simulink model "bp"  (Simulink 7.1)
settings: Solver=ode5  StartTime=0.0  StopTime=170.0  FixedStep=0.1  RelTol=1e-3  AbsTol=1e-3
undefined symbols (not defined in the file): sfunyst
libraries: fuzblock x3
settings Model: Creator=Slavi  LastModifiedBy=Slavi  BufferReuse=off
settings DataIOCC: LimitDataPoints=off  SaveOutput=off  SaveTime=off  SignalLoggingName=sigsOut
settings OptimizationCC: BlockReduction=off  BooleanDataType=off  OptimizeBlockIOStorage=off  BufferReuse=off  ExpressionFolding=off  LocalBlockOutputs=off
settings DebuggingCC: SaveWithParameterizedLinksMsg=none  SignalResolutionControl=TryResolveAllWithWarning  SolverPrmCheckMsg=none  MultiTaskDSMMsg=warning  MultiTaskCondExecSysMsg=none  StrictBusMsg=None
settings HardwareCC: TargetUnknown=on
settings RTWCC: IncludeERTFirstTime=on

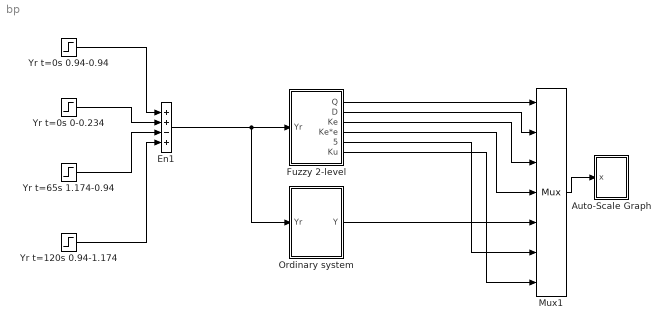
== system bp ==
  Auto-Scale Graph : Subsystem  mask(Storage scope.){@1=170, @2=0, @3=2, @4=20000, @5='r-/m-/b-/g-/k-/r-/b:', @6=.1}
      mask prompts: @1 "Initial Time Range:"; @2 "Initial y-min:"; @3 "Initial y-max:"; @4 "Storage pts.:"; @5 "Line type (rgbw-.:xo):"; @6 "Sample time:"
      mask help:
      | Storage scope using MATLAB graph window.
      | Enter plotting ranges and line type.
      mask init:
      | npts = @4; color = @5; ax = [0, @1, @2, @3]; dt=@6;
      mask Help: Uses MATLAB's graph window.\nUse only one block per system.\nLine type must be in quotes.\nSee the M-file sfunyst.m.
      mask Display: plot(0,0,100,100,[83,76,63,52,42,38,28,16,11,84,11,11,11,90,90,11],[75,58,47,54,72,80,84,74,65,65,65,90,40,40,90,90])
  En1 : Sum  Inputs=++-+  OutDataType=sfix(16)  OutScaling=2^0  SaturateOnIntegerOverflow=on  InputSameDT=on  OutDataTypeStr=Inherit: Same as first input
  Fuzzy 2-level : Subsystem
  Mux1 : Mux  Inputs=7
  Ordinary system : Subsystem
  Yr t=0s 0-0.234 : Step  Time=0  After=0.234  SampleTime=0.1
  Yr t=0s 0.94-0.94 : Step  Time=0  Before=0.94  After=0.94  SampleTime=0.1
  Yr t=120s 0.94-1.174 : Step  Time=120  After=0.234  SampleTime=0.1
  Yr t=65s 1.174-0.94 : Step  Time=65  After=0.234  SampleTime=0.1
  wires:
  Mux1/1 -> Auto-Scale Graph/1(x)
  Yr t=0s 0.94-0.94/1 -> En1/1
  En1/1 -> Fuzzy 2-level/1(Yr), Ordinary system/1(Yr)
  Fuzzy 2-level/1(Q) -> Mux1/1
  Fuzzy 2-level/2(D) -> Mux1/2
  Fuzzy 2-level/3(Ke) -> Mux1/3
  Ordinary system/1(Y) -> Mux1/5
  Fuzzy 2-level/4(Ke*e) -> Mux1/4
  Fuzzy 2-level/5("  Sum(e^2) ") -> Mux1/6
  Fuzzy 2-level/6(Ku) -> Mux1/7
  Yr t=0s 0-0.234/1 -> En1/2
  Yr t=65s 1.174-0.94/1 -> En1/3
  Yr t=120s 0.94-1.174/1 -> En1/4

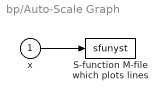
== system bp/Auto-Scale Graph ==
  x : Inport  OutDataType=sfix(16)  OutScaling=2^0
  "S-function M-file which plots lines " : S-Function  LoadFcn=sfunyst([],[],[],'LoadBlock')  FunctionName=sfunyst  Parameters=ax, color, npts, dt  EnableBusSupport=off
      settings: CopyFcn=sfunyst([],[],[],'CopyBlock')  DeleteFcn=sfunyst([],[],[],'DeleteBlock')
  wires:
  x/1 -> "S-function M-file which plots lines "/1

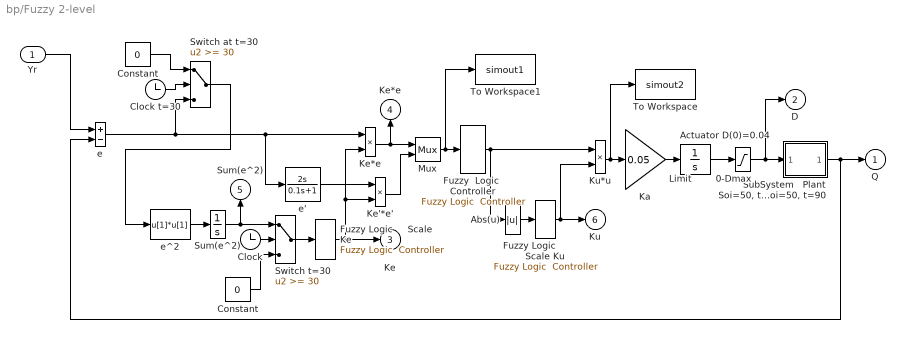
== system bp/Fuzzy 2-level ==
  Yr : Inport  SampleTime=0.5  OutDataType=sfix(16)  OutScaling=2^0
  "        Fuzzy Logic            Scale Ku" : fuzblock/Fuzzy Logic  Controller  SystemSampleTime=-1  fis=supervisor_razmit.fis
  "      Limit        0-Dmax" : Saturate  UpperLimit=0.3  LowerLimit=0
  "  Fuzzy Logic     Scale Ke" : fuzblock/Fuzzy Logic  Controller  SystemSampleTime=-1  fis=supervisor_razmit.fis
  "Abs(u) " : Abs  SaturateOnIntegerOverflow=on
  Actuator D(0)=0.04 : Integrator  InitialCondition=0.04
  Clock t=30 : Clock
      settings: Decimation=30
  "Clock  " : Clock
      settings: Decimation=30
  Constant : Constant  Value=0  OutDataType=sfix(16)  OutScaling=2^0
  "Constant " : Constant  Value=0  OutDataType=sfix(16)  OutScaling=2^0
  Fuzzy  Logic  Controller : fuzblock/Fuzzy Logic  Controller  SystemSampleTime=-1  fis=razmit_pi.fis
  Ka : Gain  Gain=0.05  ParameterDataType=sfix(16)  ParameterScaling=2^0  OutDataType=sfix(16)  OutScaling=2^0  SaturateOnIntegerOverflow=on  OutDataTypeStr=Inherit: Same as input  ParamDataTypeStr=Inherit: Same as input
  Ke'*e' : Product  OutDataType=sfix(16)  OutScaling=2^0  SaturateOnIntegerOverflow=on  InputSameDT=on  OutDataTypeStr=Inherit: Same as first input
  "Ke*e " : Product  OutDataType=sfix(16)  OutScaling=2^0  SaturateOnIntegerOverflow=on  InputSameDT=on  OutDataTypeStr=Inherit: Same as first input
  Ku*u : Product  OutDataType=sfix(16)  OutScaling=2^0  SaturateOnIntegerOverflow=on  InputSameDT=on  OutDataTypeStr=Inherit: Same as first input
  Mux : Mux  Inputs=2
  "SubSystem   Plant Soi=50, t=0 Soi=70, t=30 Soi=50, t=90" : Subsystem
  "Sum(e^2)  " : Integrator
  Switch at t=30 : Switch  Threshold=30  SaturateOnIntegerOverflow=on  InputSameDT=on
  Switch t=30 : Switch  Threshold=30  SaturateOnIntegerOverflow=on  InputSameDT=on
  To Workspace : ToWorkspace  VariableName=simout2  SampleTime=-1  SaveFormat=Array
  To Workspace1 : ToWorkspace  VariableName=simout1  SampleTime=-1  SaveFormat=Array
  e : Sum  Inputs=+-  OutDataType=sfix(16)  OutScaling=2^0  SaturateOnIntegerOverflow=on  InputSameDT=on  OutDataTypeStr=Inherit: Same as first input
  e' : TransferFcn  Numerator=[2 0]  Denominator=[0.1 1]
  e^2 : Fcn  Expr=u[1]*u[1]
  Q : Outport
  D : Outport  Port=2
  Ke : Outport  Port=3
  Ke*e : Outport  Orientation=up  Port=4
  "  Sum(e^2) " : Outport  Orientation=up  Port=5
  Ku : Outport  Port=6
  wires:
  Yr/1 -> e/1
  "SubSystem   Plant Soi=50, t=0 Soi=70, t=30 Soi=50, t=90"/1(Out2) -> Q/1, e/2
  "Ke*e "/1 -> Ke*e/1, Mux/1
  "      Limit        0-Dmax"/1 -> "SubSystem   Plant Soi=50, t=0 Soi=70, t=30 Soi=50, t=90"/1(In1), D/1
  Actuator D(0)=0.04/1 -> "      Limit        0-Dmax"/1
  Mux/1 -> Fuzzy  Logic  Controller/1, To Workspace1/1
  "  Fuzzy Logic     Scale Ke"/1 -> Ke/1, Ke'*e'/2, "Ke*e "/2
  Fuzzy  Logic  Controller/1 -> "Abs(u) "/1, Ku*u/1
  "Abs(u) "/1 -> "        Fuzzy Logic            Scale Ku"/1
  Ka/1 -> Actuator D(0)=0.04/1
  Ku*u/1 -> Ka/1, To Workspace/1
  "        Fuzzy Logic            Scale Ku"/1 -> Ku*u/2, Ku/1
  e/1 -> "Ke*e "/1, e'/1, Switch at t=30/3
  e^2/1 -> "Sum(e^2)  "/1
  "Clock  "/1 -> Switch t=30/2
  Switch t=30/1 -> "  Fuzzy Logic     Scale Ke"/1
  "Sum(e^2)  "/1 -> Switch t=30/1, "  Sum(e^2) "/1
  Constant/1 -> Switch t=30/3
  Clock t=30/1 -> Switch at t=30/2
  Switch at t=30/1 -> e^2/1
  "Constant "/1 -> Switch at t=30/1
  e'/1 -> Ke'*e'/1
  Ke'*e'/1 -> Mux/2

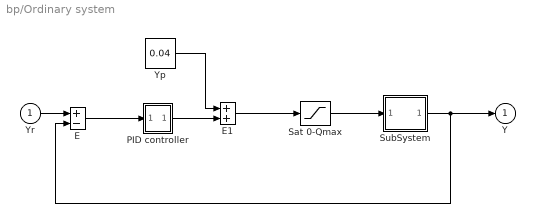
== system bp/Ordinary system ==
  Yr : Inport  SampleTime=0.5  OutDataType=sfix(16)  OutScaling=2^0
  E : Sum  Inputs=+-  OutDataType=sfix(16)  OutScaling=2^0  SaturateOnIntegerOverflow=on  InputSameDT=on  OutDataTypeStr=Inherit: Same as first input
  E1 : Sum  OutDataType=sfix(16)  OutScaling=2^0  SaturateOnIntegerOverflow=on  InputSameDT=on  OutDataTypeStr=Inherit: Same as first input
  PID controller : Subsystem  mask(PID Controller){@1=0.019, @2=0.019/1.723, @3=0}
      mask prompts: @1 "Proportional:"; @2 "Integral"; @3 "Derivative:"
      mask help:
      | Enter expressions for proportional, integral, and derivative terms.
      | P+I/s+Ds
      mask init:
      | P=@1; I=@2; D=@3;
      mask Help: This block implements a PID controller where parameters are entered for the Proportional, Integral and Derivative terms. Unmask this block to see how it works. The derivative term is implemented using a true derivative block.
      mask Display: disp('PID')
  Sat 0-Qmax : Saturate  UpperLimit=0.3  LowerLimit=0
  SubSystem : Subsystem
  Yp : Constant  Value=0.04  OutDataType=sfix(16)  OutScaling=2^0
  Y : Outport
  wires:
  E/1 -> PID controller/1(In_1)
  Yr/1 -> E/1
  SubSystem/1(Out2) -> Y/1, E/2
  Yp/1 -> E1/1
  PID controller/1(Out_1) -> E1/2
  E1/1 -> Sat 0-Qmax/1
  Sat 0-Qmax/1 -> SubSystem/1(In1)

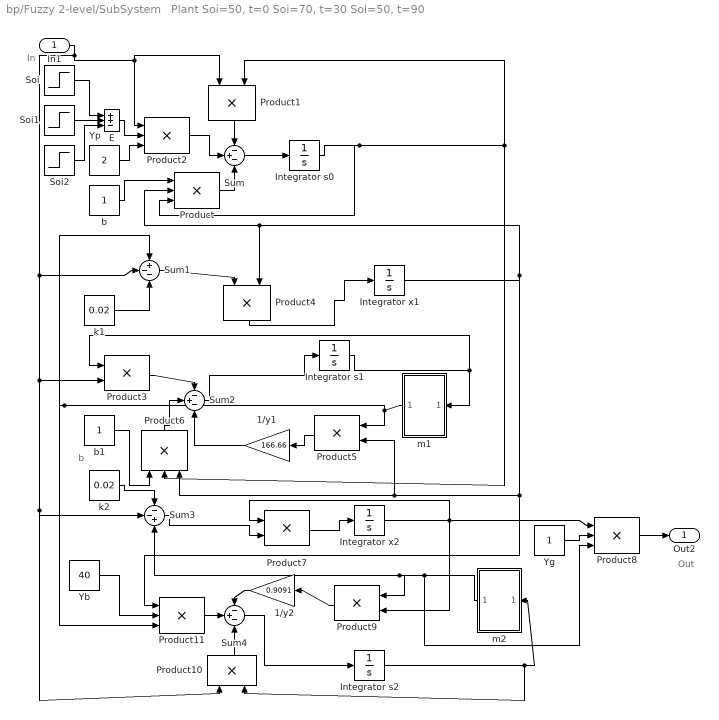
== system bp/Fuzzy 2-level/SubSystem   Plant Soi=50, t=0 Soi=70, t=30 Soi=50, t=90 ==
  note: b
  note: Out
  note: In
  In1 : Inport  OutDataType=sfix(16)  OutScaling=2^0
  1/y1 : Gain  Orientation=left  Gain=166.66  ParameterDataType=sfix(16)  ParameterScaling=2^0  OutDataType=sfix(16)  OutScaling=2^0  SaturateOnIntegerOverflow=on  OutDataTypeStr=Inherit: Same as input  ParamDataTypeStr=Inherit: Same as input
  1/y2 : Gain  Orientation=left  Gain=0.9091  ParameterDataType=sfix(16)  ParameterScaling=2^0  OutDataType=sfix(16)  OutScaling=2^0  SaturateOnIntegerOverflow=on  OutDataTypeStr=Inherit: Same as input  ParamDataTypeStr=Inherit: Same as input
  E : Sum  Inputs=++-  OutDataType=sfix(16)  OutScaling=2^0  SaturateOnIntegerOverflow=on  InputSameDT=on  OutDataTypeStr=Inherit: Same as first input
  Integrator s0 : Integrator  InitialCondition=10
  Integrator s1 : Integrator  InitialCondition=0.18
  Integrator s2 : Integrator  InitialCondition=0.18
  Integrator x1 : Integrator  InitialCondition=0.36
  Integrator x2 : Integrator  InitialCondition=15.66
  Product{,2,8,11} (4 alike) : Product  Inputs=3  OutDataType=sfix(16)  OutScaling=2^0  SaturateOnIntegerOverflow=on  InputSameDT=on  OutDataTypeStr=Inherit: Same as first input
  Product1 : Product  Orientation=down  OutDataType=sfix(16)  OutScaling=2^0  SaturateOnIntegerOverflow=on  InputSameDT=on  OutDataTypeStr=Inherit: Same as first input
  Product10 : Product  Orientation=up  OutDataType=sfix(16)  OutScaling=2^0  SaturateOnIntegerOverflow=on  InputSameDT=on  OutDataTypeStr=Inherit: Same as first input
  Product3 : Product  OutDataType=sfix(16)  OutScaling=2^0  SaturateOnIntegerOverflow=on  InputSameDT=on  OutDataTypeStr=Inherit: Same as first input
  Product4 : Product  Orientation=down  OutDataType=sfix(16)  OutScaling=2^0  SaturateOnIntegerOverflow=on  InputSameDT=on  OutDataTypeStr=Inherit: Same as first input
  Product5 : Product  Orientation=left  OutDataType=sfix(16)  OutScaling=2^0  SaturateOnIntegerOverflow=on  InputSameDT=on  OutDataTypeStr=Inherit: Same as first input
  Product6 : Product  Orientation=up  Inputs=3  OutDataType=sfix(16)  OutScaling=2^0  SaturateOnIntegerOverflow=on  InputSameDT=on  OutDataTypeStr=Inherit: Same as first input
  Product7 : Product  OutDataType=sfix(16)  OutScaling=2^0  SaturateOnIntegerOverflow=on  InputSameDT=on  OutDataTypeStr=Inherit: Same as first input
  Product9 : Product  Orientation=left  OutDataType=sfix(16)  OutScaling=2^0  SaturateOnIntegerOverflow=on  InputSameDT=on  OutDataTypeStr=Inherit: Same as first input
  Soi : Step  Time=0  Before=50  After=50  SampleTime=0.1
  Soi1 : Step  Time=30  After=20  SampleTime=0.1
  Soi2 : Step  Time=90  After=20  SampleTime=0.1
  Sum : Sum  Inputs=-+-  OutDataType=sfix(16)  OutScaling=2^0  SaturateOnIntegerOverflow=on  InputSameDT=on  OutDataTypeStr=Inherit: Same as first input
  Sum1 : Sum  Inputs=+--  OutDataType=sfix(16)  OutScaling=2^0  SaturateOnIntegerOverflow=on  InputSameDT=on  OutDataTypeStr=Inherit: Same as first input
  Sum2 : Sum  Inputs=-+-  OutDataType=sfix(16)  OutScaling=2^0  SaturateOnIntegerOverflow=on  InputSameDT=on  OutDataTypeStr=Inherit: Same as first input
  Sum3 : Sum  Inputs=--+  OutDataType=sfix(16)  OutScaling=2^0  SaturateOnIntegerOverflow=on  InputSameDT=on  OutDataTypeStr=Inherit: Same as first input
  Sum4 : Sum  Inputs=-+-  OutDataType=sfix(16)  OutScaling=2^0  SaturateOnIntegerOverflow=on  InputSameDT=on  OutDataTypeStr=Inherit: Same as first input
  Yb : Constant  Value=40  OutDataType=sfix(16)  OutScaling=2^0
  Yg : Constant  OutDataType=sfix(16)  OutScaling=2^0
  Yp : Constant  Value=2  OutDataType=sfix(16)  OutScaling=2^0
  b : Constant  OutDataType=sfix(16)  OutScaling=2^0
  b1 : Constant  OutDataType=sfix(16)  OutScaling=2^0
  k1 : Constant  Value=0.02  OutDataType=sfix(16)  OutScaling=2^0
  k2 : Constant  Value=0.02  OutDataType=sfix(16)  OutScaling=2^0
  m1 : Subsystem  Orientation=left
  m2 : Subsystem  Orientation=left
  Out2 : Outport
  wires:
  Product2/1 -> Sum/2
  Sum/1 -> Integrator s0/1
  Integrator s0/1 -> Product1/2, Product6/2, Product/3
  b/1 -> Product/1
  Sum1/1 -> Product4/1
  Product3/1 -> Sum2/1
  Product5/1 -> 1/y1/1
  Sum2/1 -> Integrator s1/1
  Product6/1 -> Sum2/2
  b1/1 -> Product6/1
  k2/1 -> Sum3/1
  Sum3/1 -> Product7/2
  Yg/1 -> Product8/2
  Product9/1 -> 1/y2/1
  m2/1(Out1) -> Product8/3, Product9/1, Sum3/3
  1/y2/1 -> Sum4/1
  Product11/1 -> Sum4/2
  Sum4/1 -> Integrator s2/1
  Integrator s1/1 -> m1/1(In1), Product3/1
  Integrator s2/1 -> Product10/2, m2/1(In1)
  Product4/1 -> Integrator x1/1
  Product1/1 -> Sum/1
  Yb/1 -> Product11/2
  m1/1(Out1) -> Product5/1, Sum1/1, Product11/3
  Integrator x1/1 -> Product5/2, Product6/3, Product11/1, Product/2, Product4/2
  Product8/1 -> Out2/1
  In1/1 -> Product1/1, Product2/1, Product10/1, Sum3/2, Product3/2, Sum1/2
  Product7/1 -> Integrator x2/1
  Integrator x2/1 -> Product8/1, Product9/2, Product7/1
  Product/1 -> Sum/3
  k1/1 -> Sum1/3
  Product10/1 -> Sum4/3
  1/y1/1 -> Sum2/3
  Yp/1 -> Product2/3
  E/1 -> Product2/2
  Soi1/1 -> E/2
  Soi/1 -> E/1
  Soi2/1 -> E/3

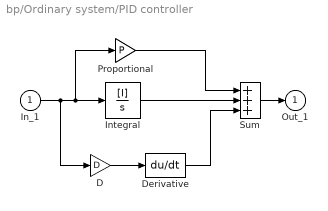
== system bp/Ordinary system/PID controller ==
  In_1 : Inport  OutDataType=sfix(16)  OutScaling=2^0
  D : Gain  Gain=D  ParameterDataType=sfix(16)  ParameterScaling=2^0  OutDataType=sfix(16)  OutScaling=2^0  SaturateOnIntegerOverflow=on  OutDataTypeStr=Inherit: Same as input  ParamDataTypeStr=Inherit: Same as input
  Derivative : Derivative
  Integral : TransferFcn  Numerator=[I]  Denominator=[1 0]
  Proportional : Gain  Gain=P  ParameterDataType=sfix(16)  ParameterScaling=2^0  OutDataType=sfix(16)  OutScaling=2^0  SaturateOnIntegerOverflow=on  OutDataTypeStr=Inherit: Same as input  ParamDataTypeStr=Inherit: Same as input
  Sum : Sum  Inputs=+++  OutDataType=sfix(16)  OutScaling=2^0  SaturateOnIntegerOverflow=on  InputSameDT=on  OutDataTypeStr=Inherit: Same as first input
  Out_1 : Outport
  wires:
  D/1 -> Derivative/1
  Sum/1 -> Out_1/1
  In_1/1 -> D/1, Integral/1, Proportional/1
  Integral/1 -> Sum/2
  Proportional/1 -> Sum/1
  Derivative/1 -> Sum/3

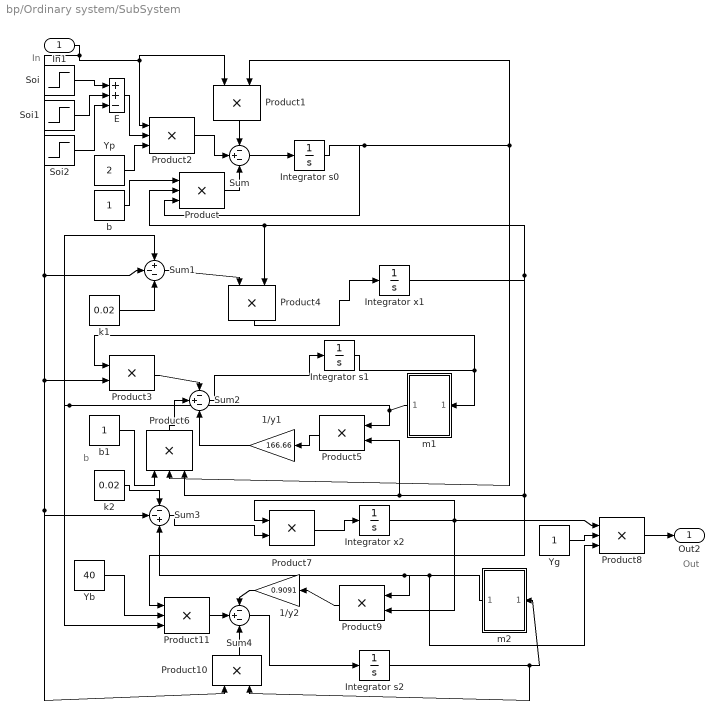
== system bp/Ordinary system/SubSystem ==
  note: b
  note: Out
  note: In
  In1 : Inport  OutDataType=sfix(16)  OutScaling=2^0
  1/y1 : Gain  Orientation=left  Gain=166.66  ParameterDataType=sfix(16)  ParameterScaling=2^0  OutDataType=sfix(16)  OutScaling=2^0  SaturateOnIntegerOverflow=on  OutDataTypeStr=Inherit: Same as input  ParamDataTypeStr=Inherit: Same as input
  1/y2 : Gain  Orientation=left  Gain=0.9091  ParameterDataType=sfix(16)  ParameterScaling=2^0  OutDataType=sfix(16)  OutScaling=2^0  SaturateOnIntegerOverflow=on  OutDataTypeStr=Inherit: Same as input  ParamDataTypeStr=Inherit: Same as input
  E : Sum  Inputs=++-  OutDataType=sfix(16)  OutScaling=2^0  SaturateOnIntegerOverflow=on  InputSameDT=on  OutDataTypeStr=Inherit: Same as first input
  Integrator s0 : Integrator  InitialCondition=10
  Integrator s1 : Integrator  InitialCondition=0.18
  Integrator s2 : Integrator  InitialCondition=0.18
  Integrator x1 : Integrator  InitialCondition=0.36
  Integrator x2 : Integrator  InitialCondition=15.66
  Product{,2,8,11} (4 alike) : Product  Inputs=3  OutDataType=sfix(16)  OutScaling=2^0  SaturateOnIntegerOverflow=on  InputSameDT=on  OutDataTypeStr=Inherit: Same as first input
  Product1 : Product  Orientation=down  OutDataType=sfix(16)  OutScaling=2^0  SaturateOnIntegerOverflow=on  InputSameDT=on  OutDataTypeStr=Inherit: Same as first input
  Product10 : Product  Orientation=up  OutDataType=sfix(16)  OutScaling=2^0  SaturateOnIntegerOverflow=on  InputSameDT=on  OutDataTypeStr=Inherit: Same as first input
  Product3 : Product  OutDataType=sfix(16)  OutScaling=2^0  SaturateOnIntegerOverflow=on  InputSameDT=on  OutDataTypeStr=Inherit: Same as first input
  Product4 : Product  Orientation=down  OutDataType=sfix(16)  OutScaling=2^0  SaturateOnIntegerOverflow=on  InputSameDT=on  OutDataTypeStr=Inherit: Same as first input
  Product5 : Product  Orientation=left  OutDataType=sfix(16)  OutScaling=2^0  SaturateOnIntegerOverflow=on  InputSameDT=on  OutDataTypeStr=Inherit: Same as first input
  Product6 : Product  Orientation=up  Inputs=3  OutDataType=sfix(16)  OutScaling=2^0  SaturateOnIntegerOverflow=on  InputSameDT=on  OutDataTypeStr=Inherit: Same as first input
  Product7 : Product  OutDataType=sfix(16)  OutScaling=2^0  SaturateOnIntegerOverflow=on  InputSameDT=on  OutDataTypeStr=Inherit: Same as first input
  Product9 : Product  Orientation=left  OutDataType=sfix(16)  OutScaling=2^0  SaturateOnIntegerOverflow=on  InputSameDT=on  OutDataTypeStr=Inherit: Same as first input
  Soi : Step  Time=0  Before=50  After=50  SampleTime=0.1
  Soi1 : Step  Time=30  After=20  SampleTime=0.1
  Soi2 : Step  Time=90  After=20  SampleTime=0.1
  Sum : Sum  Inputs=-+-  OutDataType=sfix(16)  OutScaling=2^0  SaturateOnIntegerOverflow=on  InputSameDT=on  OutDataTypeStr=Inherit: Same as first input
  Sum1 : Sum  Inputs=+--  OutDataType=sfix(16)  OutScaling=2^0  SaturateOnIntegerOverflow=on  InputSameDT=on  OutDataTypeStr=Inherit: Same as first input
  Sum2 : Sum  Inputs=-+-  OutDataType=sfix(16)  OutScaling=2^0  SaturateOnIntegerOverflow=on  InputSameDT=on  OutDataTypeStr=Inherit: Same as first input
  Sum3 : Sum  Inputs=--+  OutDataType=sfix(16)  OutScaling=2^0  SaturateOnIntegerOverflow=on  InputSameDT=on  OutDataTypeStr=Inherit: Same as first input
  Sum4 : Sum  Inputs=-+-  OutDataType=sfix(16)  OutScaling=2^0  SaturateOnIntegerOverflow=on  InputSameDT=on  OutDataTypeStr=Inherit: Same as first input
  Yb : Constant  Value=40  OutDataType=sfix(16)  OutScaling=2^0
  Yg : Constant  OutDataType=sfix(16)  OutScaling=2^0
  Yp : Constant  Value=2  OutDataType=sfix(16)  OutScaling=2^0
  b : Constant  OutDataType=sfix(16)  OutScaling=2^0
  b1 : Constant  OutDataType=sfix(16)  OutScaling=2^0
  k1 : Constant  Value=0.02  OutDataType=sfix(16)  OutScaling=2^0
  k2 : Constant  Value=0.02  OutDataType=sfix(16)  OutScaling=2^0
  m1 : Subsystem  Orientation=left
  m2 : Subsystem  Orientation=left
  Out2 : Outport
  wires:
  Product2/1 -> Sum/2
  Sum/1 -> Integrator s0/1
  Integrator s0/1 -> Product1/2, Product6/2, Product/3
  b/1 -> Product/1
  Sum1/1 -> Product4/1
  Product3/1 -> Sum2/1
  Product5/1 -> 1/y1/1
  Sum2/1 -> Integrator s1/1
  Product6/1 -> Sum2/2
  b1/1 -> Product6/1
  k2/1 -> Sum3/1
  Sum3/1 -> Product7/2
  Yg/1 -> Product8/2
  Product9/1 -> 1/y2/1
  m2/1(Out1) -> Product8/3, Product9/1, Sum3/3
  1/y2/1 -> Sum4/1
  Product11/1 -> Sum4/2
  Sum4/1 -> Integrator s2/1
  Integrator s1/1 -> m1/1(In1), Product3/1
  Integrator s2/1 -> Product10/2, m2/1(In1)
  Product4/1 -> Integrator x1/1
  Product1/1 -> Sum/1
  Yb/1 -> Product11/2
  m1/1(Out1) -> Product5/1, Sum1/1, Product11/3
  Integrator x1/1 -> Product5/2, Product6/3, Product11/1, Product/2, Product4/2
  Product8/1 -> Out2/1
  In1/1 -> Product1/1, Product2/1, Product10/1, Sum3/2, Product3/2, Sum1/2
  Product7/1 -> Integrator x2/1
  Integrator x2/1 -> Product8/1, Product9/2, Product7/1
  Product/1 -> Sum/3
  k1/1 -> Sum1/3
  Product10/1 -> Sum4/3
  1/y1/1 -> Sum2/3
  Yp/1 -> Product2/3
  Soi/1 -> E/1
  Soi1/1 -> E/2
  E/1 -> Product2/2
  Soi2/1 -> E/3

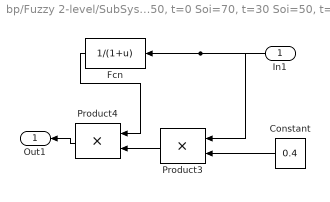
== system bp/Fuzzy 2-level/SubSystem   Plant Soi=50, t=0 Soi=70, t=30 Soi=50, t=90/m1 ==
  In1 : Inport  Orientation=left  OutDataType=sfix(16)  OutScaling=2^0
  Constant : Constant  Orientation=left  Value=0.4  OutDataType=sfix(16)  OutScaling=2^0
  Fcn : Fcn  Orientation=left  Expr=1/(1+u)
  Product3 : Product  Orientation=left  OutDataType=sfix(16)  OutScaling=2^0  SaturateOnIntegerOverflow=on  InputSameDT=on  OutDataTypeStr=Inherit: Same as first input
  Product4 : Product  Orientation=left  OutDataType=sfix(16)  OutScaling=2^0  SaturateOnIntegerOverflow=on  InputSameDT=on  OutDataTypeStr=Inherit: Same as first input
  Out1 : Outport  Orientation=left
  wires:
  In1/1 -> Product3/1, Fcn/1
  Product3/1 -> Product4/2
  Product4/1 -> Out1/1
  Fcn/1 -> Product4/1
  Constant/1 -> Product3/2

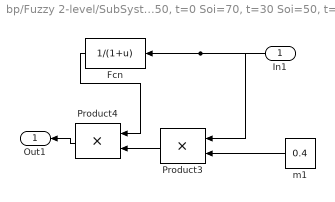
== system bp/Fuzzy 2-level/SubSystem   Plant Soi=50, t=0 Soi=70, t=30 Soi=50, t=90/m2 ==
  In1 : Inport  Orientation=left  OutDataType=sfix(16)  OutScaling=2^0
  Fcn : Fcn  Orientation=left  Expr=1/(1+u)
  Product3 : Product  Orientation=left  OutDataType=sfix(16)  OutScaling=2^0  SaturateOnIntegerOverflow=on  InputSameDT=on  OutDataTypeStr=Inherit: Same as first input
  Product4 : Product  Orientation=left  OutDataType=sfix(16)  OutScaling=2^0  SaturateOnIntegerOverflow=on  InputSameDT=on  OutDataTypeStr=Inherit: Same as first input
  m1 : Constant  Orientation=left  Value=0.4  OutDataType=sfix(16)  OutScaling=2^0
  Out1 : Outport  Orientation=left
  wires:
  In1/1 -> Product3/1, Fcn/1
  m1/1 -> Product3/2
  Product3/1 -> Product4/2
  Product4/1 -> Out1/1
  Fcn/1 -> Product4/1

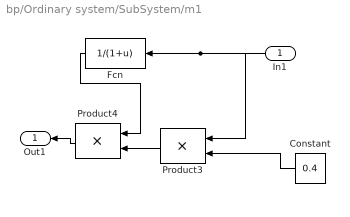
== system bp/Ordinary system/SubSystem/m1 ==
  In1 : Inport  Orientation=left  OutDataType=sfix(16)  OutScaling=2^0
  Constant : Constant  Orientation=left  Value=0.4  OutDataType=sfix(16)  OutScaling=2^0
  Fcn : Fcn  Orientation=left  Expr=1/(1+u)
  Product3 : Product  Orientation=left  OutDataType=sfix(16)  OutScaling=2^0  SaturateOnIntegerOverflow=on  InputSameDT=on  OutDataTypeStr=Inherit: Same as first input
  Product4 : Product  Orientation=left  OutDataType=sfix(16)  OutScaling=2^0  SaturateOnIntegerOverflow=on  InputSameDT=on  OutDataTypeStr=Inherit: Same as first input
  Out1 : Outport  Orientation=left
  wires:
  In1/1 -> Product3/1, Fcn/1
  Constant/1 -> Product3/2
  Product3/1 -> Product4/2
  Product4/1 -> Out1/1
  Fcn/1 -> Product4/1

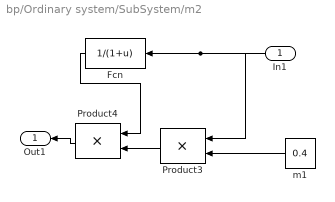
== system bp/Ordinary system/SubSystem/m2 ==
  In1 : Inport  Orientation=left  OutDataType=sfix(16)  OutScaling=2^0
  Fcn : Fcn  Orientation=left  Expr=1/(1+u)
  Product3 : Product  Orientation=left  OutDataType=sfix(16)  OutScaling=2^0  SaturateOnIntegerOverflow=on  InputSameDT=on  OutDataTypeStr=Inherit: Same as first input
  Product4 : Product  Orientation=left  OutDataType=sfix(16)  OutScaling=2^0  SaturateOnIntegerOverflow=on  InputSameDT=on  OutDataTypeStr=Inherit: Same as first input
  m1 : Constant  Orientation=left  Value=0.4  OutDataType=sfix(16)  OutScaling=2^0
  Out1 : Outport  Orientation=left
  wires:
  In1/1 -> Product3/1, Fcn/1
  m1/1 -> Product3/2
  Product3/1 -> Product4/2
  Product4/1 -> Out1/1
  Fcn/1 -> Product4/1
